simulink model "ground_vehicle_sim"  (R2021a)
settings: Solver=VariableStepAuto  StartTime=0.0  StopTime=200  FixedStep=0.0001  RelTol=1e-9
values from neighbouring files (symbols this model uses):
  framePeriod_s = 1/frameRate_hz    (= 0.02)    [autocode_setup.m]    (also in config.m; setup.m)
undefined symbols (not defined in the file or in its folder): Aircraft, datetime, datevec, Earth, Env, Fmu, InitCond, Telem, WGS84
libraries: simulink x8, aerolibconvert2 x5, aerolibasang x3, aerolibtransform2 x2, aerolibgravity2 x2, aerolibatmos2 x1, sharedtransform x1, uavutilslib x1, shared6dof x1
(part 3 of 3)

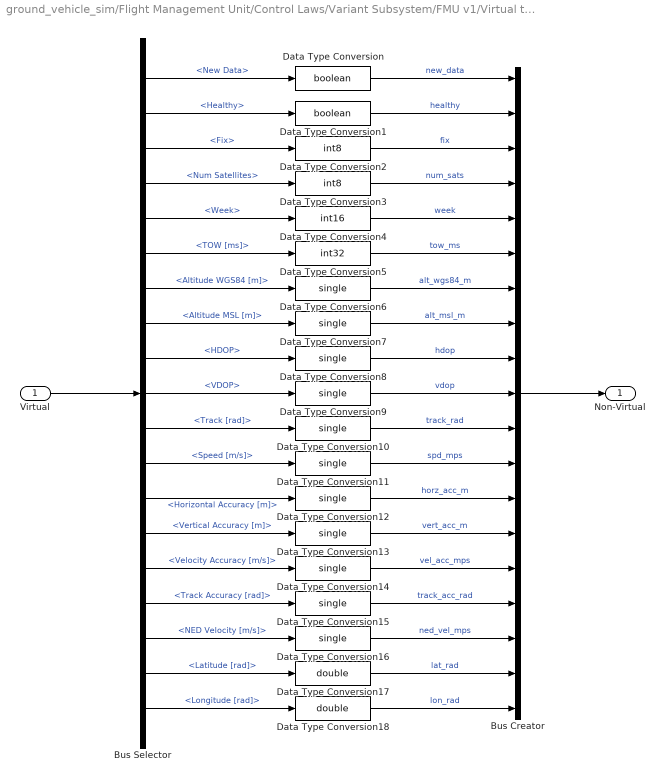
== system ground_vehicle_sim/Flight Management Unit/Control Laws/Variant Subsystem/FMU v1/Virtual to Non-Virtual Mapping1/Virtual to Non-Virtual Mapping3 ==
  Virtual : Inport
  Bus Creator : BusCreator  Inputs=19
  Bus Selector : BusSelector  OutputSignals=New Data,Healthy,Fix,Num Satellites,Week,TOW [ms],Altitude WGS84 [m],Altitude MSL [m],HDOP,VDOP,Track [rad],Speed [m/s],Horizontal Accuracy [m],Vertical Accuracy [m],Velocity Accuracy [m/s],Track Accuracy [rad],NED Velocity [m/s],Latitude [rad],Longitude [rad]
  Data Type Conversion : DataTypeConversion  OutDataTypeStr=boolean
  Data Type Conversion1 : DataTypeConversion  OutDataTypeStr=boolean
  Data Type Conversion{6..16} (11 alike) : DataTypeConversion  OutDataTypeStr=single
  Data Type Conversion17 : DataTypeConversion  OutDataTypeStr=double
  Data Type Conversion18 : DataTypeConversion  OutDataTypeStr=double
  Data Type Conversion2 : DataTypeConversion  OutDataTypeStr=int8
  Data Type Conversion3 : DataTypeConversion  OutDataTypeStr=int8
  Data Type Conversion4 : DataTypeConversion  OutDataTypeStr=int16
  Data Type Conversion5 : DataTypeConversion  OutDataTypeStr=int32
  Non-Virtual : Outport  OutDataTypeStr=Bus: GnssData
  wires:
  Data Type Conversion12/1 -> Bus Creator/13  "horz_acc_m"
  Data Type Conversion13/1 -> Bus Creator/14  "vert_acc_m"
  Data Type Conversion14/1 -> Bus Creator/15  "vel_acc_mps"
  Data Type Conversion15/1 -> Bus Creator/16  "track_acc_rad"
  Data Type Conversion16/1 -> Bus Creator/17  "ned_vel_mps"
  Data Type Conversion17/1 -> Bus Creator/18  "lat_rad"
  Data Type Conversion18/1 -> Bus Creator/19  "lon_rad"
  Bus Selector/19 -> Data Type Conversion18/1  "<Longitude [rad]>"
  Bus Selector/18 -> Data Type Conversion17/1  "<Latitude [rad]>"
  Bus Selector/17 -> Data Type Conversion16/1  "<NED Velocity [m/s]>"
  Bus Selector/16 -> Data Type Conversion15/1  "<Track Accuracy [rad]>"
  Bus Selector/15 -> Data Type Conversion14/1  "<Velocity Accuracy [m/s]>"
  Bus Selector/14 -> Data Type Conversion13/1  "<Vertical Accuracy [m]>"
  Bus Selector/13 -> Data Type Conversion12/1  "<Horizontal Accuracy [m]>"
  Data Type Conversion11/1 -> Bus Creator/12  "spd_mps"
  Data Type Conversion10/1 -> Bus Creator/11  "track_rad"
  Bus Selector/12 -> Data Type Conversion11/1  "<Speed [m/s]>"
  Bus Selector/11 -> Data Type Conversion10/1  "<Track [rad]>"
  Data Type Conversion9/1 -> Bus Creator/10  "vdop"
  Data Type Conversion8/1 -> Bus Creator/9  "hdop"
  Bus Selector/10 -> Data Type Conversion9/1  "<VDOP>"
  Bus Selector/9 -> Data Type Conversion8/1  "<HDOP>"
  Data Type Conversion7/1 -> Bus Creator/8  "alt_msl_m"
  Data Type Conversion6/1 -> Bus Creator/7  "alt_wgs84_m"
  Bus Selector/8 -> Data Type Conversion7/1  "<Altitude MSL [m]>"
  Bus Selector/7 -> Data Type Conversion6/1  "<Altitude WGS84 [m]>"
  Data Type Conversion5/1 -> Bus Creator/6  "tow_ms"
  Bus Selector/6 -> Data Type Conversion5/1  "<TOW [ms]>"
  Data Type Conversion4/1 -> Bus Creator/5  "week"
  Bus Selector/5 -> Data Type Conversion4/1  "<Week>"
  Data Type Conversion3/1 -> Bus Creator/4  "num_sats"
  Bus Selector/4 -> Data Type Conversion3/1  "<Num Satellites>"
  Data Type Conversion2/1 -> Bus Creator/3  "fix"
  Bus Selector/3 -> Data Type Conversion2/1  "<Fix>"
  Data Type Conversion1/1 -> Bus Creator/2  "healthy"
  Bus Selector/2 -> Data Type Conversion1/1  "<Healthy>"
  Data Type Conversion/1 -> Bus Creator/1  "new_data"
  Bus Selector/1 -> Data Type Conversion/1  "<New Data>"
  Bus Creator/1 -> Non-Virtual/1
  Virtual/1 -> Bus Selector/1

== system ground_vehicle_sim/Flight Management Unit/Control Laws/Variant Subsystem/FMU v1/Virtual to Non-Virtual Mapping1/Virtual to Non-Virtual Mapping4 ==
  Virtual : Inport
  Bus Creator : BusCreator  Inputs=4
  Bus Selector : BusSelector  OutputSignals=New Data,Healthy,Pressure [Pa],Die Temperature [C]
  Data Type Conversion : DataTypeConversion  OutDataTypeStr=boolean
  Data Type Conversion1 : DataTypeConversion  OutDataTypeStr=boolean
  Data Type Conversion2 : DataTypeConversion  OutDataTypeStr=single
  Data Type Conversion3 : DataTypeConversion  OutDataTypeStr=single
  Non-Virtual : Outport  OutDataTypeStr=Bus: PresData
  wires:
  Data Type Conversion3/1 -> Bus Creator/4  "die_temp_c"
  Bus Selector/4 -> Data Type Conversion3/1  "<Die Temperature [C]>"
  Data Type Conversion2/1 -> Bus Creator/3  "pres_pa"
  Bus Selector/3 -> Data Type Conversion2/1  "<Pressure [Pa]>"
  Data Type Conversion1/1 -> Bus Creator/2  "healthy"
  Bus Selector/2 -> Data Type Conversion1/1  "<Healthy>"
  Data Type Conversion/1 -> Bus Creator/1  "new_data"
  Bus Selector/1 -> Data Type Conversion/1  "<New Data>"
  Virtual/1 -> Bus Selector/1
  Bus Creator/1 -> Non-Virtual/1

== system ground_vehicle_sim/Flight Management Unit/Control Laws/Variant Subsystem/FMU v1/Virtual to Non-Virtual Mapping1/Virtual to Non-Virtual Mapping5 ==
  Virtual : Inport
  Bus Creator : BusCreator  Inputs=4
  Bus Selector : BusSelector  OutputSignals=New Data,Healthy,Pressure [Pa],Die Temperature [C]
  Data Type Conversion : DataTypeConversion  OutDataTypeStr=boolean
  Data Type Conversion1 : DataTypeConversion  OutDataTypeStr=boolean
  Data Type Conversion2 : DataTypeConversion  OutDataTypeStr=single
  Data Type Conversion3 : DataTypeConversion  OutDataTypeStr=single
  Non-Virtual : Outport  OutDataTypeStr=Bus: PresData
  wires:
  Bus Creator/1 -> Non-Virtual/1
  Virtual/1 -> Bus Selector/1
  Bus Selector/1 -> Data Type Conversion/1  "<New Data>"
  Data Type Conversion/1 -> Bus Creator/1  "new_data"
  Bus Selector/2 -> Data Type Conversion1/1  "<Healthy>"
  Data Type Conversion1/1 -> Bus Creator/2  "healthy"
  Bus Selector/3 -> Data Type Conversion2/1  "<Pressure [Pa]>"
  Data Type Conversion2/1 -> Bus Creator/3  "pres_pa"
  Bus Selector/4 -> Data Type Conversion3/1  "<Die Temperature [C]>"
  Data Type Conversion3/1 -> Bus Creator/4  "die_temp_c"

== system ground_vehicle_sim/Flight Management Unit/Control Laws/Variant Subsystem/FMU v1/Virtual to Non-Virtual Mapping1/Virtual to Non-Virtual Mapping6 ==
  Virtual : Inport
  Bus Creator : BusCreator  Inputs=2
  Bus Selector : BusSelector  OutputSignals=Voltages,Values
  Data Type Conversion2 : DataTypeConversion  OutDataTypeStr=single
  Data Type Conversion3 : DataTypeConversion  OutDataTypeStr=single
  Non-Virtual : Outport  OutDataTypeStr=Bus: AnalogData
  wires:
  Data Type Conversion3/1 -> Bus Creator/2  "val"
  Bus Selector/2 -> Data Type Conversion3/1  "<Values>"
  Bus Selector/1 -> Data Type Conversion2/1  "<Voltages>"
  Data Type Conversion2/1 -> Bus Creator/1  "volt"
  Virtual/1 -> Bus Selector/1
  Bus Creator/1 -> Non-Virtual/1

== system ground_vehicle_sim/Flight Management Unit/Control Laws/Variant Subsystem/FMU v2/Virtual to Non-Virtual Mapping4/Subsystem1 ==
  Non-Virtual : Inport  OutDataTypeStr=Bus: BatteryData
  Bus Creator : BusCreator  Inputs=5
  Bus Selector : BusSelector  OutputSignals=voltage_v,current_ma,consumed_mah,remaining_prcnt,remaining_time_s
  Data Type Conversion{,1..4} (5 alike) : DataTypeConversion  OutDataTypeStr=double
  Virtual : Outport
  wires:
  Non-Virtual/1 -> Bus Selector/1
  Bus Selector/1 -> Data Type Conversion/1  "<voltage_v>"
  Bus Selector/2 -> Data Type Conversion1/1  "<current_ma>"
  Bus Selector/3 -> Data Type Conversion2/1  "<consumed_mah>"
  Bus Selector/4 -> Data Type Conversion3/1  "<remaining_prcnt>"
  Bus Selector/5 -> Data Type Conversion4/1  "<remaining_time_s>"
  Bus Creator/1 -> Virtual/1
  Data Type Conversion/1 -> Bus Creator/1  "Voltage [V]"
  Data Type Conversion1/1 -> Bus Creator/2  "Current [mA]"
  Data Type Conversion2/1 -> Bus Creator/3  "Consumed Capacity [mAh]"
  Data Type Conversion3/1 -> Bus Creator/4  "Remaining Capacity [%]"
  Data Type Conversion4/1 -> Bus Creator/5  "Remaining Flight Time [s]"

== system ground_vehicle_sim/Flight Management Unit/Control Laws/Variant Subsystem/FMU v2/Virtual to Non-Virtual Mapping4/Subsystem2 ==
  Non-Virtual : Inport  OutDataTypeStr=Bus: AnalogData
  Bus Creator : BusCreator  Inputs=1
  Bus Selector : BusSelector  OutputSignals=val
  Data Type Conversion : DataTypeConversion  OutDataTypeStr=double
  Virtual : Outport
  wires:
  Non-Virtual/1 -> Bus Selector/1
  Bus Creator/1 -> Virtual/1
  Data Type Conversion/1 -> Bus Creator/1  "Values"
  Bus Selector/1 -> Data Type Conversion/1  "<val>"

== system ground_vehicle_sim/Flight Management Unit/Control Laws/Variant Subsystem/FMU v2/Virtual to Non-Virtual Mapping4/Subsystem3 ==
  Non-Virtual : Inport  OutDataTypeStr=Bus: PwmCmd
  Bus Creator : BusCreator  Inputs=2
  Bus Selector : BusSelector  OutputSignals=cnt,cmd
  Data Type Conversion : DataTypeConversion  OutDataTypeStr=double
  Data Type Conversion1 : DataTypeConversion  OutDataTypeStr=double
  Virtual : Outport
  wires:
  Non-Virtual/1 -> Bus Selector/1
  Bus Selector/2 -> Data Type Conversion1/1  "<cmd>"
  Data Type Conversion1/1 -> Bus Creator/2  "Cmds"
  Data Type Conversion/1 -> Bus Creator/1  "Cnt"
  Bus Selector/1 -> Data Type Conversion/1  "<cnt>"
  Bus Creator/1 -> Virtual/1

== system ground_vehicle_sim/Flight Management Unit/Control Laws/Variant Subsystem/FMU v2/Virtual to Non-Virtual Mapping4/Subsystem4 ==
  Non-Virtual : Inport  OutDataTypeStr=Bus: SbusCmd
  Bus Creator : BusCreator  Inputs=4
  Bus Selector : BusSelector  OutputSignals=ch17,ch18,cnt,cmd
  Data Type Conversion{,1..3} (4 alike) : DataTypeConversion  OutDataTypeStr=double
  Virtual : Outport
  wires:
  Non-Virtual/1 -> Bus Selector/1
  Bus Creator/1 -> Virtual/1
  Bus Selector/1 -> Data Type Conversion/1  "<ch17>"
  Bus Selector/2 -> Data Type Conversion1/1  "<ch18>"
  Bus Selector/3 -> Data Type Conversion2/1  "<cnt>"
  Bus Selector/4 -> Data Type Conversion3/1  "<cmd>"
  Data Type Conversion2/1 -> Bus Creator/3  "Cnt"
  Data Type Conversion3/1 -> Bus Creator/4  "Cmds"
  Data Type Conversion1/1 -> Bus Creator/2  "Ch 18"
  Data Type Conversion/1 -> Bus Creator/1  "Ch 17"

== system ground_vehicle_sim/Flight Management Unit/Control Laws/Variant Subsystem/FMU v2/Virtual to Non-Virtual Mapping5/Virtual to Non-Virtual Mapping1 ==
  Virtual : Inport
  Bus Creator : BusCreator  Inputs=6
  Bus Selector : BusSelector  OutputSignals=New Data,Lost Frame,Failsafe,Ch 17,Ch 18,Channel Data
  Data Type Conversion{,1..4} (5 alike) : DataTypeConversion  OutDataTypeStr=boolean
  Data Type Conversion5 : DataTypeConversion  OutDataTypeStr=int16
  Non-Virtual : Outport  OutDataTypeStr=Bus: InceptorData
  wires:
  Virtual/1 -> Bus Selector/1
  Bus Creator/1 -> Non-Virtual/1
  Bus Selector/1 -> Data Type Conversion/1  "<New Data>"
  Bus Selector/2 -> Data Type Conversion1/1  "<Lost Frame>"
  Bus Selector/3 -> Data Type Conversion2/1  "<Failsafe>"
  Bus Selector/4 -> Data Type Conversion3/1  "<Ch 17>"
  Bus Selector/5 -> Data Type Conversion4/1  "<Ch 18>"
  Bus Selector/6 -> Data Type Conversion5/1  "<Channel Data>"
  Data Type Conversion/1 -> Bus Creator/1  "new_data"
  Data Type Conversion1/1 -> Bus Creator/2  "lost_frame"
  Data Type Conversion2/1 -> Bus Creator/3  "failsafe"
  Data Type Conversion3/1 -> Bus Creator/4  "ch17"
  Data Type Conversion4/1 -> Bus Creator/5  "ch18"
  Data Type Conversion5/1 -> Bus Creator/6  "ch"

== system ground_vehicle_sim/Flight Management Unit/Control Laws/Variant Subsystem/FMU v2/Virtual to Non-Virtual Mapping5/Virtual to Non-Virtual Mapping2 ==
  Virtual : Inport
  Bus Creator : BusCreator  Inputs=8
  Bus Selector : BusSelector  OutputSignals=New IMU Data,New Magnetometer Data,IMU Healthy,Magnetometer Healthy,Die Temperature [C],Accelerometer [m/s/s],Gyro [rad/s],Magnetometer [uT]
  Data Type Conversion{,1..3} (4 alike) : DataTypeConversion  OutDataTypeStr=boolean
  Data Type Conversion{4..7} (4 alike) : DataTypeConversion  OutDataTypeStr=single
  Non-Virtual : Outport  OutDataTypeStr=Bus: ImuData
  wires:
  Bus Creator/1 -> Non-Virtual/1
  Virtual/1 -> Bus Selector/1
  Bus Selector/1 -> Data Type Conversion/1  "<New IMU Data>"
  Data Type Conversion/1 -> Bus Creator/1  "new_imu_data"
  Bus Selector/2 -> Data Type Conversion1/1  "<New Magnetometer Data>"
  Data Type Conversion1/1 -> Bus Creator/2  "new_mag_data"
  Bus Selector/3 -> Data Type Conversion2/1  "<IMU Healthy>"
  Data Type Conversion2/1 -> Bus Creator/3  "imu_healthy"
  Bus Selector/4 -> Data Type Conversion3/1  "<Magnetometer Healthy>"
  Data Type Conversion3/1 -> Bus Creator/4  "mag_healthy"
  Bus Selector/5 -> Data Type Conversion4/1  "<Die Temperature [C]>"
  Data Type Conversion4/1 -> Bus Creator/5  "die_temp_c"
  Bus Selector/6 -> Data Type Conversion5/1  "<Accelerometer [m/s/s]>"
  Bus Selector/7 -> Data Type Conversion6/1  "<Gyro [rad/s]>"
  Bus Selector/8 -> Data Type Conversion7/1  "<Magnetometer [uT]>"
  Data Type Conversion5/1 -> Bus Creator/6  "accel_mps2"
  Data Type Conversion6/1 -> Bus Creator/7  "gyro_radps"
  Data Type Conversion7/1 -> Bus Creator/8  "mag_ut"

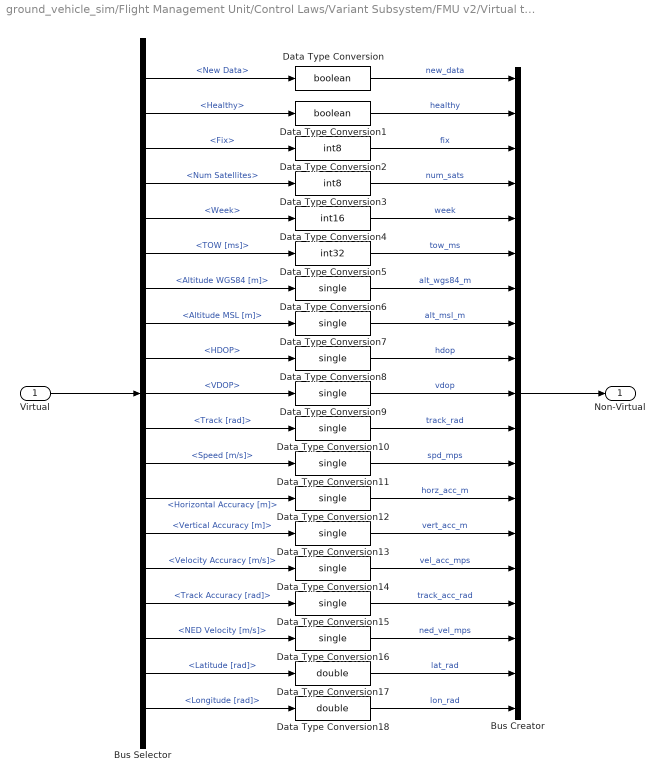
== system ground_vehicle_sim/Flight Management Unit/Control Laws/Variant Subsystem/FMU v2/Virtual to Non-Virtual Mapping5/Virtual to Non-Virtual Mapping3 ==
  Virtual : Inport
  Bus Creator : BusCreator  Inputs=19
  Bus Selector : BusSelector  OutputSignals=New Data,Healthy,Fix,Num Satellites,Week,TOW [ms],Altitude WGS84 [m],Altitude MSL [m],HDOP,VDOP,Track [rad],Speed [m/s],Horizontal Accuracy [m],Vertical Accuracy [m],Velocity Accuracy [m/s],Track Accuracy [rad],NED Velocity [m/s],Latitude [rad],Longitude [rad]
  Data Type Conversion : DataTypeConversion  OutDataTypeStr=boolean
  Data Type Conversion1 : DataTypeConversion  OutDataTypeStr=boolean
  Data Type Conversion{6..16} (11 alike) : DataTypeConversion  OutDataTypeStr=single
  Data Type Conversion17 : DataTypeConversion  OutDataTypeStr=double
  Data Type Conversion18 : DataTypeConversion  OutDataTypeStr=double
  Data Type Conversion2 : DataTypeConversion  OutDataTypeStr=int8
  Data Type Conversion3 : DataTypeConversion  OutDataTypeStr=int8
  Data Type Conversion4 : DataTypeConversion  OutDataTypeStr=int16
  Data Type Conversion5 : DataTypeConversion  OutDataTypeStr=int32
  Non-Virtual : Outport  OutDataTypeStr=Bus: GnssData
  wires:
  Virtual/1 -> Bus Selector/1
  Bus Creator/1 -> Non-Virtual/1
  Bus Selector/1 -> Data Type Conversion/1  "<New Data>"
  Data Type Conversion/1 -> Bus Creator/1  "new_data"
  Bus Selector/2 -> Data Type Conversion1/1  "<Healthy>"
  Data Type Conversion1/1 -> Bus Creator/2  "healthy"
  Bus Selector/3 -> Data Type Conversion2/1  "<Fix>"
  Data Type Conversion2/1 -> Bus Creator/3  "fix"
  Bus Selector/4 -> Data Type Conversion3/1  "<Num Satellites>"
  Data Type Conversion3/1 -> Bus Creator/4  "num_sats"
  Bus Selector/5 -> Data Type Conversion4/1  "<Week>"
  Data Type Conversion4/1 -> Bus Creator/5  "week"
  Bus Selector/6 -> Data Type Conversion5/1  "<TOW [ms]>"
  Data Type Conversion5/1 -> Bus Creator/6  "tow_ms"
  Bus Selector/7 -> Data Type Conversion6/1  "<Altitude WGS84 [m]>"
  Bus Selector/8 -> Data Type Conversion7/1  "<Altitude MSL [m]>"
  Data Type Conversion6/1 -> Bus Creator/7  "alt_wgs84_m"
  Data Type Conversion7/1 -> Bus Creator/8  "alt_msl_m"
  Bus Selector/9 -> Data Type Conversion8/1  "<HDOP>"
  Bus Selector/10 -> Data Type Conversion9/1  "<VDOP>"
  Data Type Conversion8/1 -> Bus Creator/9  "hdop"
  Data Type Conversion9/1 -> Bus Creator/10  "vdop"
  Bus Selector/11 -> Data Type Conversion10/1  "<Track [rad]>"
  Bus Selector/12 -> Data Type Conversion11/1  "<Speed [m/s]>"
  Data Type Conversion10/1 -> Bus Creator/11  "track_rad"
  Data Type Conversion11/1 -> Bus Creator/12  "spd_mps"
  Bus Selector/13 -> Data Type Conversion12/1  "<Horizontal Accuracy [m]>"
  Bus Selector/14 -> Data Type Conversion13/1  "<Vertical Accuracy [m]>"
  Bus Selector/15 -> Data Type Conversion14/1  "<Velocity Accuracy [m/s]>"
  Bus Selector/16 -> Data Type Conversion15/1  "<Track Accuracy [rad]>"
  Bus Selector/17 -> Data Type Conversion16/1  "<NED Velocity [m/s]>"
  Bus Selector/18 -> Data Type Conversion17/1  "<Latitude [rad]>"
  Bus Selector/19 -> Data Type Conversion18/1  "<Longitude [rad]>"
  Data Type Conversion18/1 -> Bus Creator/19  "lon_rad"
  Data Type Conversion17/1 -> Bus Creator/18  "lat_rad"
  Data Type Conversion16/1 -> Bus Creator/17  "ned_vel_mps"
  Data Type Conversion15/1 -> Bus Creator/16  "track_acc_rad"
  Data Type Conversion14/1 -> Bus Creator/15  "vel_acc_mps"
  Data Type Conversion13/1 -> Bus Creator/14  "vert_acc_m"
  Data Type Conversion12/1 -> Bus Creator/13  "horz_acc_m"

== system ground_vehicle_sim/Flight Management Unit/Control Laws/Variant Subsystem/FMU v2/Virtual to Non-Virtual Mapping5/Virtual to Non-Virtual Mapping4 ==
  Virtual : Inport
  Bus Creator : BusCreator  Inputs=4
  Bus Selector : BusSelector  OutputSignals=New Data,Healthy,Pressure [Pa],Die Temperature [C]
  Data Type Conversion : DataTypeConversion  OutDataTypeStr=boolean
  Data Type Conversion1 : DataTypeConversion  OutDataTypeStr=boolean
  Data Type Conversion2 : DataTypeConversion  OutDataTypeStr=single
  Data Type Conversion3 : DataTypeConversion  OutDataTypeStr=single
  Non-Virtual : Outport  OutDataTypeStr=Bus: PresData
  wires:
  Bus Creator/1 -> Non-Virtual/1
  Virtual/1 -> Bus Selector/1
  Bus Selector/1 -> Data Type Conversion/1  "<New Data>"
  Data Type Conversion/1 -> Bus Creator/1  "new_data"
  Bus Selector/2 -> Data Type Conversion1/1  "<Healthy>"
  Data Type Conversion1/1 -> Bus Creator/2  "healthy"
  Bus Selector/3 -> Data Type Conversion2/1  "<Pressure [Pa]>"
  Data Type Conversion2/1 -> Bus Creator/3  "pres_pa"
  Bus Selector/4 -> Data Type Conversion3/1  "<Die Temperature [C]>"
  Data Type Conversion3/1 -> Bus Creator/4  "die_temp_c"

== system ground_vehicle_sim/Flight Management Unit/Control Laws/Variant Subsystem/FMU v2/Virtual to Non-Virtual Mapping5/Virtual to Non-Virtual Mapping5 ==
  Virtual : Inport
  Bus Creator : BusCreator  Inputs=4
  Bus Selector : BusSelector  OutputSignals=New Data,Healthy,Pressure [Pa],Die Temperature [C]
  Data Type Conversion : DataTypeConversion  OutDataTypeStr=boolean
  Data Type Conversion1 : DataTypeConversion  OutDataTypeStr=boolean
  Data Type Conversion2 : DataTypeConversion  OutDataTypeStr=single
  Data Type Conversion3 : DataTypeConversion  OutDataTypeStr=single
  Non-Virtual : Outport  OutDataTypeStr=Bus: PresData
  wires:
  Data Type Conversion3/1 -> Bus Creator/4  "die_temp_c"
  Bus Selector/4 -> Data Type Conversion3/1  "<Die Temperature [C]>"
  Data Type Conversion2/1 -> Bus Creator/3  "pres_pa"
  Bus Selector/3 -> Data Type Conversion2/1  "<Pressure [Pa]>"
  Data Type Conversion1/1 -> Bus Creator/2  "healthy"
  Bus Selector/2 -> Data Type Conversion1/1  "<Healthy>"
  Data Type Conversion/1 -> Bus Creator/1  "new_data"
  Bus Selector/1 -> Data Type Conversion/1  "<New Data>"
  Virtual/1 -> Bus Selector/1
  Bus Creator/1 -> Non-Virtual/1

== system ground_vehicle_sim/Flight Management Unit/Control Laws/Variant Subsystem/FMU v2/Virtual to Non-Virtual Mapping5/Virtual to Non-Virtual Mapping6 ==
  Virtual : Inport
  Bus Creator : BusCreator  Inputs=1
  Bus Selector : BusSelector  OutputSignals=Voltages
  Data Type Conversion2 : DataTypeConversion  OutDataTypeStr=single
  Non-Virtual : Outport  OutDataTypeStr=Bus: AdcData
  wires:
  Bus Creator/1 -> Non-Virtual/1
  Virtual/1 -> Bus Selector/1
  Data Type Conversion2/1 -> Bus Creator/1  "volt"
  Bus Selector/1 -> Data Type Conversion2/1  "<Voltages>"

== system ground_vehicle_sim/Flight Management Unit/Control Laws/Variant Subsystem/FMU v2/Virtual to Non-Virtual Mapping5/Virtual to Non-Virtual Mapping7 ==
  Virtual : Inport
  Bus Creator : BusCreator  Inputs=2
  Bus Selector : BusSelector  OutputSignals=Voltage [V],Current [V]
  Data Type Conversion1 : DataTypeConversion  OutDataTypeStr=single
  Data Type Conversion2 : DataTypeConversion  OutDataTypeStr=single
  Non-Virtual : Outport  OutDataTypeStr=Bus: PowerModuleData
  wires:
  Virtual/1 -> Bus Selector/1
  Bus Creator/1 -> Non-Virtual/1
  Bus Selector/1 -> Data Type Conversion1/1  "<Voltage [V]>"
  Data Type Conversion1/1 -> Bus Creator/1  "voltage_v"
  Bus Selector/2 -> Data Type Conversion2/1  "<Current [V]>"
  Data Type Conversion2/1 -> Bus Creator/2  "current_v"

== system ground_vehicle_sim/Flight Management Unit/Control Laws/Variant Subsystem/FMU v2 Beta/Virtual to Non-Virtual Mapping1/Virtual to Non-Virtual Mapping1 ==
  Virtual : Inport
  Bus Creator : BusCreator  Inputs=10
  Bus Selector : BusSelector  OutputSignals=New Data,Lost Frame,Failsafe,Throttle Enable,Mode 0,Mode 1,Throttle,Pitch,Pitch,Yaw
  Data Type Conversion{,1..3} (4 alike) : DataTypeConversion  OutDataTypeStr=boolean
  Data Type Conversion4 : DataTypeConversion  OutDataTypeStr=int8
  Data Type Conversion5 : DataTypeConversion  OutDataTypeStr=int8
  Data Type Conversion{6..9} (4 alike) : DataTypeConversion  OutDataTypeStr=single
  Non-Virtual : Outport  OutDataTypeStr=Bus: InceptorData
  wires:
  Virtual/1 -> Bus Selector/1
  Bus Creator/1 -> Non-Virtual/1
  Bus Selector/1 -> Data Type Conversion/1  "<New Data>"
  Data Type Conversion/1 -> Bus Creator/1  "new_data"
  Bus Selector/2 -> Data Type Conversion1/1  "<Lost Frame>"
  Bus Selector/3 -> Data Type Conversion2/1  "<Failsafe>"
  Bus Selector/4 -> Data Type Conversion3/1  "<Throttle Enable>"
  Bus Selector/5 -> Data Type Conversion4/1  "<Mode 0>"
  Bus Selector/6 -> Data Type Conversion5/1  "<Mode 1>"
  Bus Selector/7 -> Data Type Conversion6/1  "<Throttle>"
  Bus Selector/8 -> Data Type Conversion7/1  "<Pitch>"
  Bus Selector/9 -> Data Type Conversion8/1  "<Pitch>"
  Bus Selector/10 -> Data Type Conversion9/1  "<Yaw>"
  Data Type Conversion1/1 -> Bus Creator/2  "lost_frame"
  Data Type Conversion2/1 -> Bus Creator/3  "failsafe"
  Data Type Conversion3/1 -> Bus Creator/4  "throttle_en"
  Data Type Conversion4/1 -> Bus Creator/5  "mode0"
  Data Type Conversion5/1 -> Bus Creator/6  "mode1"
  Data Type Conversion6/1 -> Bus Creator/7  "throttle"
  Data Type Conversion7/1 -> Bus Creator/8  "pitch"
  Data Type Conversion8/1 -> Bus Creator/9  "roll"
  Data Type Conversion9/1 -> Bus Creator/10  "yaw"

== system ground_vehicle_sim/Flight Management Unit/Control Laws/Variant Subsystem/FMU v2 Beta/Virtual to Non-Virtual Mapping1/Virtual to Non-Virtual Mapping2 ==
  Virtual : Inport
  Bus Creator : BusCreator  Inputs=8
  Bus Selector : BusSelector  OutputSignals=New IMU Data,New Magnetometer Data,IMU Healthy,Magnetometer Healthy,Die Temperature [C],Accelerometer [m/s/s],Gyro [rad/s],Magnetometer [uT]
  Data Type Conversion{,1..3} (4 alike) : DataTypeConversion  OutDataTypeStr=boolean
  Data Type Conversion{4..7} (4 alike) : DataTypeConversion  OutDataTypeStr=single
  Non-Virtual : Outport  OutDataTypeStr=Bus: ImuData
  wires:
  Bus Creator/1 -> Non-Virtual/1
  Virtual/1 -> Bus Selector/1
  Bus Selector/1 -> Data Type Conversion/1  "<New IMU Data>"
  Data Type Conversion/1 -> Bus Creator/1  "new_imu_data"
  Bus Selector/2 -> Data Type Conversion1/1  "<New Magnetometer Data>"
  Data Type Conversion1/1 -> Bus Creator/2  "new_mag_data"
  Bus Selector/3 -> Data Type Conversion2/1  "<IMU Healthy>"
  Data Type Conversion2/1 -> Bus Creator/3  "imu_healthy"
  Bus Selector/4 -> Data Type Conversion3/1  "<Magnetometer Healthy>"
  Data Type Conversion3/1 -> Bus Creator/4  "mag_healthy"
  Bus Selector/5 -> Data Type Conversion4/1  "<Die Temperature [C]>"
  Data Type Conversion4/1 -> Bus Creator/5  "die_temp_c"
  Bus Selector/6 -> Data Type Conversion5/1  "<Accelerometer [m/s/s]>"
  Bus Selector/7 -> Data Type Conversion6/1  "<Gyro [rad/s]>"
  Bus Selector/8 -> Data Type Conversion7/1  "<Magnetometer [uT]>"
  Data Type Conversion5/1 -> Bus Creator/6  "accel_mps2"
  Data Type Conversion6/1 -> Bus Creator/7  "gyro_radps"
  Data Type Conversion7/1 -> Bus Creator/8  "mag_ut"

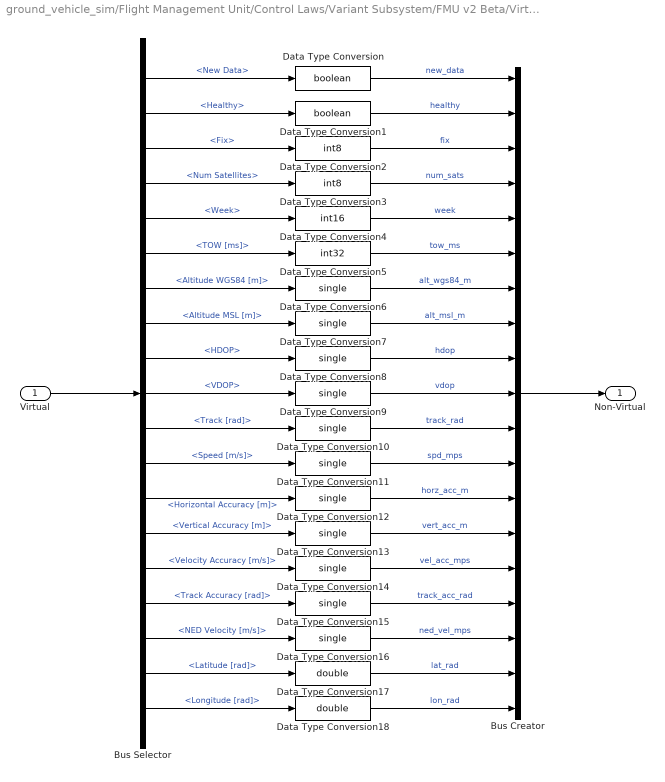
== system ground_vehicle_sim/Flight Management Unit/Control Laws/Variant Subsystem/FMU v2 Beta/Virtual to Non-Virtual Mapping1/Virtual to Non-Virtual Mapping3 ==
  Virtual : Inport
  Bus Creator : BusCreator  Inputs=19
  Bus Selector : BusSelector  OutputSignals=New Data,Healthy,Fix,Num Satellites,Week,TOW [ms],Altitude WGS84 [m],Altitude MSL [m],HDOP,VDOP,Track [rad],Speed [m/s],Horizontal Accuracy [m],Vertical Accuracy [m],Velocity Accuracy [m/s],Track Accuracy [rad],NED Velocity [m/s],Latitude [rad],Longitude [rad]
  Data Type Conversion : DataTypeConversion  OutDataTypeStr=boolean
  Data Type Conversion1 : DataTypeConversion  OutDataTypeStr=boolean
  Data Type Conversion{6..16} (11 alike) : DataTypeConversion  OutDataTypeStr=single
  Data Type Conversion17 : DataTypeConversion  OutDataTypeStr=double
  Data Type Conversion18 : DataTypeConversion  OutDataTypeStr=double
  Data Type Conversion2 : DataTypeConversion  OutDataTypeStr=int8
  Data Type Conversion3 : DataTypeConversion  OutDataTypeStr=int8
  Data Type Conversion4 : DataTypeConversion  OutDataTypeStr=int16
  Data Type Conversion5 : DataTypeConversion  OutDataTypeStr=int32
  Non-Virtual : Outport  OutDataTypeStr=Bus: GnssData
  wires:
  Virtual/1 -> Bus Selector/1
  Bus Creator/1 -> Non-Virtual/1
  Bus Selector/1 -> Data Type Conversion/1  "<New Data>"
  Data Type Conversion/1 -> Bus Creator/1  "new_data"
  Bus Selector/2 -> Data Type Conversion1/1  "<Healthy>"
  Data Type Conversion1/1 -> Bus Creator/2  "healthy"
  Bus Selector/3 -> Data Type Conversion2/1  "<Fix>"
  Data Type Conversion2/1 -> Bus Creator/3  "fix"
  Bus Selector/4 -> Data Type Conversion3/1  "<Num Satellites>"
  Data Type Conversion3/1 -> Bus Creator/4  "num_sats"
  Bus Selector/5 -> Data Type Conversion4/1  "<Week>"
  Data Type Conversion4/1 -> Bus Creator/5  "week"
  Bus Selector/6 -> Data Type Conversion5/1  "<TOW [ms]>"
  Data Type Conversion5/1 -> Bus Creator/6  "tow_ms"
  Bus Selector/7 -> Data Type Conversion6/1  "<Altitude WGS84 [m]>"
  Bus Selector/8 -> Data Type Conversion7/1  "<Altitude MSL [m]>"
  Data Type Conversion6/1 -> Bus Creator/7  "alt_wgs84_m"
  Data Type Conversion7/1 -> Bus Creator/8  "alt_msl_m"
  Bus Selector/9 -> Data Type Conversion8/1  "<HDOP>"
  Bus Selector/10 -> Data Type Conversion9/1  "<VDOP>"
  Data Type Conversion8/1 -> Bus Creator/9  "hdop"
  Data Type Conversion9/1 -> Bus Creator/10  "vdop"
  Bus Selector/11 -> Data Type Conversion10/1  "<Track [rad]>"
  Bus Selector/12 -> Data Type Conversion11/1  "<Speed [m/s]>"
  Data Type Conversion10/1 -> Bus Creator/11  "track_rad"
  Data Type Conversion11/1 -> Bus Creator/12  "spd_mps"
  Bus Selector/13 -> Data Type Conversion12/1  "<Horizontal Accuracy [m]>"
  Bus Selector/14 -> Data Type Conversion13/1  "<Vertical Accuracy [m]>"
  Bus Selector/15 -> Data Type Conversion14/1  "<Velocity Accuracy [m/s]>"
  Bus Selector/16 -> Data Type Conversion15/1  "<Track Accuracy [rad]>"
  Bus Selector/17 -> Data Type Conversion16/1  "<NED Velocity [m/s]>"
  Bus Selector/18 -> Data Type Conversion17/1  "<Latitude [rad]>"
  Bus Selector/19 -> Data Type Conversion18/1  "<Longitude [rad]>"
  Data Type Conversion18/1 -> Bus Creator/19  "lon_rad"
  Data Type Conversion17/1 -> Bus Creator/18  "lat_rad"
  Data Type Conversion16/1 -> Bus Creator/17  "ned_vel_mps"
  Data Type Conversion15/1 -> Bus Creator/16  "track_acc_rad"
  Data Type Conversion14/1 -> Bus Creator/15  "vel_acc_mps"
  Data Type Conversion13/1 -> Bus Creator/14  "vert_acc_m"
  Data Type Conversion12/1 -> Bus Creator/13  "horz_acc_m"

== system ground_vehicle_sim/Flight Management Unit/Control Laws/Variant Subsystem/FMU v2 Beta/Virtual to Non-Virtual Mapping1/Virtual to Non-Virtual Mapping4 ==
  Virtual : Inport
  Bus Creator : BusCreator  Inputs=4
  Bus Selector : BusSelector  OutputSignals=New Data,Healthy,Pressure [Pa],Die Temperature [C]
  Data Type Conversion : DataTypeConversion  OutDataTypeStr=boolean
  Data Type Conversion1 : DataTypeConversion  OutDataTypeStr=boolean
  Data Type Conversion2 : DataTypeConversion  OutDataTypeStr=single
  Data Type Conversion3 : DataTypeConversion  OutDataTypeStr=single
  Non-Virtual : Outport  OutDataTypeStr=Bus: PresData
  wires:
  Bus Creator/1 -> Non-Virtual/1
  Virtual/1 -> Bus Selector/1
  Bus Selector/1 -> Data Type Conversion/1  "<New Data>"
  Data Type Conversion/1 -> Bus Creator/1  "new_data"
  Bus Selector/2 -> Data Type Conversion1/1  "<Healthy>"
  Data Type Conversion1/1 -> Bus Creator/2  "healthy"
  Bus Selector/3 -> Data Type Conversion2/1  "<Pressure [Pa]>"
  Data Type Conversion2/1 -> Bus Creator/3  "pres_pa"
  Bus Selector/4 -> Data Type Conversion3/1  "<Die Temperature [C]>"
  Data Type Conversion3/1 -> Bus Creator/4  "die_temp_c"

== system ground_vehicle_sim/Flight Management Unit/Control Laws/Variant Subsystem/FMU v2 Beta/Virtual to Non-Virtual Mapping1/Virtual to Non-Virtual Mapping5 ==
  Virtual : Inport
  Bus Creator : BusCreator  Inputs=4
  Bus Selector : BusSelector  OutputSignals=New Data,Healthy,Pressure [Pa],Die Temperature [C]
  Data Type Conversion : DataTypeConversion  OutDataTypeStr=boolean
  Data Type Conversion1 : DataTypeConversion  OutDataTypeStr=boolean
  Data Type Conversion2 : DataTypeConversion  OutDataTypeStr=single
  Data Type Conversion3 : DataTypeConversion  OutDataTypeStr=single
  Non-Virtual : Outport  OutDataTypeStr=Bus: PresData
  wires:
  Data Type Conversion3/1 -> Bus Creator/4  "die_temp_c"
  Bus Selector/4 -> Data Type Conversion3/1  "<Die Temperature [C]>"
  Data Type Conversion2/1 -> Bus Creator/3  "pres_pa"
  Bus Selector/3 -> Data Type Conversion2/1  "<Pressure [Pa]>"
  Data Type Conversion1/1 -> Bus Creator/2  "healthy"
  Bus Selector/2 -> Data Type Conversion1/1  "<Healthy>"
  Data Type Conversion/1 -> Bus Creator/1  "new_data"
  Bus Selector/1 -> Data Type Conversion/1  "<New Data>"
  Virtual/1 -> Bus Selector/1
  Bus Creator/1 -> Non-Virtual/1

== system ground_vehicle_sim/Flight Management Unit/Control Laws/Variant Subsystem/FMU v2 Beta/Virtual to Non-Virtual Mapping1/Virtual to Non-Virtual Mapping6 ==
  Virtual : Inport
  Bus Creator : BusCreator  Inputs=2
  Bus Selector : BusSelector  OutputSignals=Voltages,Values
  Data Type Conversion2 : DataTypeConversion  OutDataTypeStr=single
  Data Type Conversion3 : DataTypeConversion  OutDataTypeStr=single
  Non-Virtual : Outport  OutDataTypeStr=Bus: AnalogData
  wires:
  Bus Creator/1 -> Non-Virtual/1
  Virtual/1 -> Bus Selector/1
  Data Type Conversion2/1 -> Bus Creator/1  "volt"
  Bus Selector/1 -> Data Type Conversion2/1  "<Voltages>"
  Bus Selector/2 -> Data Type Conversion3/1  "<Values>"
  Data Type Conversion3/1 -> Bus Creator/2  "val"

== matlab function ground_vehicle_sim/Vehicle/Vehicle Model/MATLAB Function ==
  data: ang input; ret output
function ret  = constrain360(ang)
%Constrain360 Converts a +/-180 value to a 0 - 360 value
ret = fmod(ang, 360);
if ret < 0
    ret = ret + 360;
end

end

== matlab function ground_vehicle_sim/Flight Management Unit/Sensor Models/GNSS/Triggered Subsystem/MATLAB Function ==
  data: year input; month input; mday input; hour input; minute input; second input; gnss_week output; sim_clock input; gnss_tow output
function [gnss_week, gnss_tow] = GnssWeekAndTime(year, month, mday, hour, minute, second, sim_clock)

JAN61980 = 44244;
JAN11901 = 15385;
SEC_PER_DAY = 86400.0;

month_day = [
    0, 31, 59, 90, 120, 151, 181, 212, 243, 273, 304, 334;
    0, 31, 60, 91, 121, 152, 182, 213, 244, 274, 305, 335
];

second = second + sim_clock;
leap = (mod(year,4) == 0);
yday = month_day(leap + 1, month) + mday;
mjd = ((year - 1901) / 4) * 1461 + mod((year - 1901), 4) * 365 + yday - 1 + JAN11901;
fmjd = ((second / 60.0 + minute) / 60.0 + hour) / 24.0;
gnss_week = floor((mjd - JAN61980) / 7);
gnss_tow = ((mjd - JAN61980) - gnss_week * 7 + fmjd) * SEC_PER_DAY;

== matlab function ground_vehicle_sim/Flight Management Unit/Sensor Models/GNSS/Triggered Subsystem/MATLAB Function1 ==
  data: ang input; ret output
function ret  = constrain360(ang)
%Constrain360 Converts a +/-180 value to a 0 - 360 value
ret = fmod(ang, 360);
if ret < 0
    ret = ret + 360;
end

end
